simulink model "wakeDeflection_th"  (R2018b)
settings: Solver=VariableStepAuto  StartTime=0.0  StopTime=0  RelTol=1e-3
values from neighbouring files (symbols this model uses):
  downstreamTurbPos = [8;0;0]    [bayesian_ts.m]    (also in wakeDeflection_ts.m = [4;0;0])
  upstreamTurbFlow = 4    [bayesian_ts.m]    (also in wakeDeflection_ts.m)
  upstreamTurbPos = [0;0;0]    [bayesian_ts.m]    (also in wakeDeflection_ts.m)
  upstreamTurbYaw = 10*pi/180    (= 0.174532925199)    [bayesian_ts.m]    (also in wakeDeflection_ts.m)
libraries: wakeDeflection_ul x1
settings Model: Creator=asiddiq2  LastModifiedBy=asiddiq2

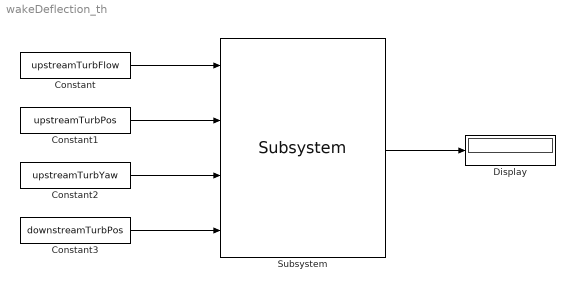
== system wakeDeflection_th ==
  Constant : Constant  Value=upstreamTurbFlow  VectorParams1D=off
  Constant1 : Constant  Value=upstreamTurbPos  VectorParams1D=off
  Constant2 : Constant  Value=upstreamTurbYaw  VectorParams1D=off
  Constant3 : Constant  Value=downstreamTurbPos  VectorParams1D=off
  Display : Display
  Subsystem : wakeDeflection_ul/Subsystem  nTheta=nth  nD=nd  turbDia=td
  wires:
  Constant/1 -> Subsystem/1
  Constant1/1 -> Subsystem/2
  Constant2/1 -> Subsystem/3
  Constant3/1 -> Subsystem/4
  Subsystem/1 -> Display/1
